simulink model "q1"  (R2021a)
settings: Solver=FixedStepAuto  StartTime=0.0  StopTime=10.0  FixedStep=0.001  RelTol=1e-3
libraries: cstblocks x7
settings Model: Creator=HASEE  LastModifiedBy=HASEE

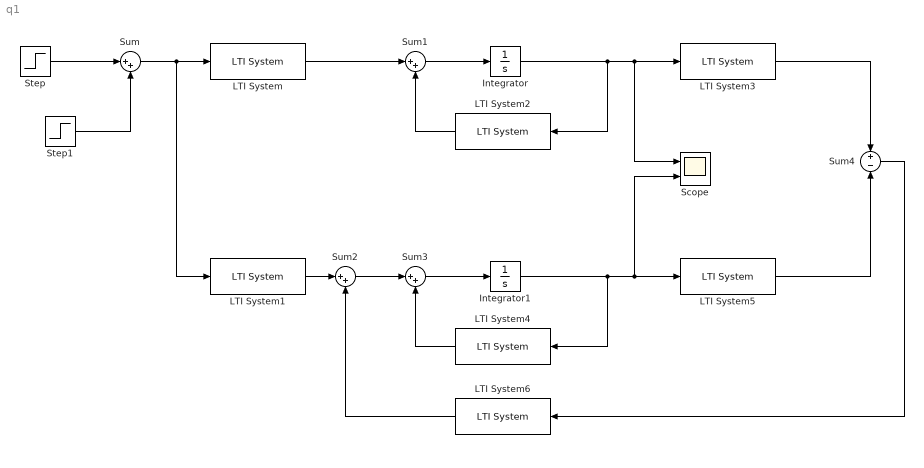
== system q1 ==
  Integrator : Integrator  InitialCondition=[pi/3 0 0 0]
  Integrator1 : Integrator
  LTI System : cstblocks/LTI System  sys=B  IC=[]
  LTI System1 : cstblocks/LTI System  sys=B  IC=[]
  LTI System2 : cstblocks/LTI System  sys=A  IC=[]
  LTI System3 : cstblocks/LTI System  sys=C2  IC=[]
  LTI System4 : cstblocks/LTI System  sys=A  IC=[]
  LTI System5 : cstblocks/LTI System  sys=C2  IC=[]
  LTI System6 : cstblocks/LTI System  sys=L2  IC=[]
  Scope : Scope  NumInputPorts=2
  Step : Step  Time=0.1  SampleTime=0
  Step1 : Step  Time=0.2  After=-1  SampleTime=0
  Sum{,1..3} (4 alike) : Sum  Inputs=|++
  Sum4 : Sum  Inputs=+|-
  wires:
  Step/1 -> Sum/1
  Step1/1 -> Sum/2
  Sum/1 -> LTI System1/1, LTI System/1
  LTI System/1 -> Sum1/1
  Sum1/1 -> Integrator/1
  Integrator/1 -> Scope/1, LTI System3/1, LTI System2/1
  LTI System2/1 -> Sum1/2
  LTI System1/1 -> Sum2/1
  Integrator1/1 -> Scope/2, LTI System5/1, LTI System4/1
  LTI System4/1 -> Sum3/2
  Sum3/1 -> Integrator1/1
  Sum2/1 -> Sum3/1
  LTI System3/1 -> Sum4/1
  LTI System5/1 -> Sum4/2
  Sum4/1 -> LTI System6/1
  LTI System6/1 -> Sum2/2
